simulink model "model2"  (R2022b)
settings: Solver=ode3  StartTime=0.0  StopTime=5  FixedStep=0.0005  RelTol=1e-3
values from neighbouring files (symbols this model uses):
  a21 = 1/2/m * x30^2 * FemP1/FemP2^2 * exp(-x10/FemP2)    [init.m]    (also in proj.m)
  a23 = -1/m * x30 * FemP1/FemP2 * exp(-x10/FemP2)    [init.m]    (also in proj.m)
  a31 = 1/f1 * exp(x10/f2) * (ki*u10 + ci - x30)    [init.m]    (also in proj.m)
  a33 = -f2/f1 * exp(x10/f2)    [init.m]    (also in proj.m)
  b31 = ki * f2/f1 * exp(x10/f2)    [init.m]    (also in proj.m)
  g = 9.81    [init.m]    (also in proj.m)
  kd = 4    [init.m]    (also in proj.m = 1)
  ki = 30    [init.m]    (also in proj.m = 0.2)
  kp = 110    [init.m]    (also in proj.m = 80)
  xd = d-bd    [init.m]    (also in proj.m)
settings Model: Creator=TheZl  LastModifiedBy=TheZl

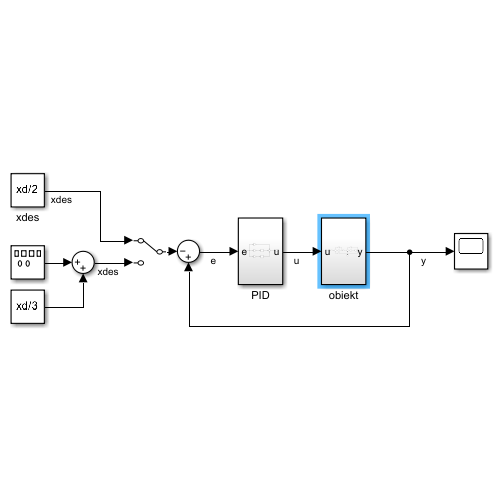
[thumbnail: Simulink's stored preview of the top-level diagram]
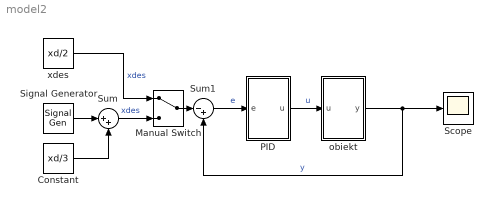
== system model2 ==
  Constant : Constant  Value=xd/3
  Manual Switch : ManualSwitch
  PID : Subsystem
  Scope : Scope
  Signal Generator : SignalGenerator  Amplitude=xd/4  Frequency=5  Units=rad/sec
  Sum : Sum  Inputs=|++
  Sum1 : Sum  Inputs=|-+
  obiekt : Subsystem
  xdes : Constant  Value=xd/2
  wires:
  obiekt/1(y) -> Scope/1, Sum1/2  "y"
  PID/1(u) -> obiekt/1(u)  "u"
  Sum1/1 -> PID/1(e)  "e"
  Signal Generator/1 -> Sum/1
  Constant/1 -> Sum/2
  Manual Switch/1 -> Sum1/1
  Sum/1 -> Manual Switch/2  "xdes"
  xdes/1 -> Manual Switch/1  "xdes"

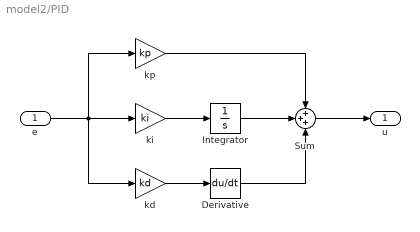
== system model2/PID ==
  e : Inport
  Derivative : Derivative
  Integrator : Integrator
  Sum : Sum  Inputs=+++
  kd : Gain  Gain=kd
  ki : Gain  Gain=ki
  kp : Gain  Gain=kp
  u : Outport
  wires:
  Integrator/1 -> Sum/2
  kd/1 -> Derivative/1
  Derivative/1 -> Sum/3
  ki/1 -> Integrator/1
  Sum/1 -> u/1
  e/1 -> ki/1, kd/1, kp/1
  kp/1 -> Sum/1

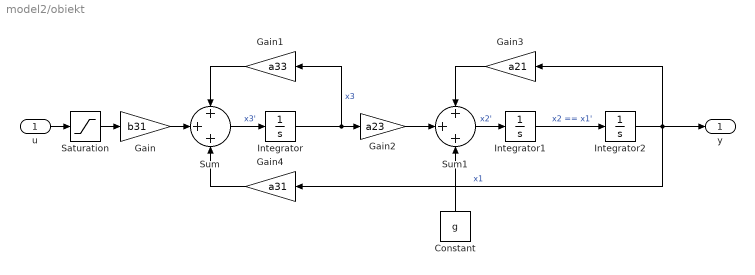
== system model2/obiekt ==
  u : Inport
  Constant : Constant  Value=g
  Gain : Gain  Gain=b31
  Gain1 : Gain  Gain=a33
  Gain2 : Gain  Gain=a23
  Gain3 : Gain  Gain=a21
  Gain4 : Gain  Gain=a31
  Integrator : Integrator
  Integrator1 : Integrator
  Integrator2 : Integrator  InitialCondition=xd  LimitOutput=on  UpperSaturationLimit=xd  LowerSaturationLimit=0
  Saturation : Saturate  UpperLimit=1  LowerLimit=0
  Sum : Sum  Inputs=+++
  Sum1 : Sum  Inputs=+++
  y : Outport
  wires:
  u/1 -> Saturation/1
  Saturation/1 -> Gain/1
  Integrator2/1 -> y/1, Gain4/1, Gain3/1  "x1"
  Constant/1 -> Sum1/3
  Gain1/1 -> Sum/1
  Sum/1 -> Integrator/1  "x3'"
  Integrator1/1 -> Integrator2/1  "x2 == x1'"
  Sum1/1 -> Integrator1/1  "x2'"
  Integrator/1 -> Gain1/1, Gain2/1  "x3"
  Gain2/1 -> Sum1/2
  Gain/1 -> Sum/2
  Gain3/1 -> Sum1/1
  Gain4/1 -> Sum/3
